simulink model "DeltaWingPlantHGO"  (R2024b)
settings: Solver=VariableStepAuto  StartTime=0.0  StopTime=60  MaxStep=0.01  RelTol=1e-3  EnableMultiTasking=on
InitFcn:
  | global Ba La gamma_a
  | beta0 = 0.4;
  | betap0 = 0;
  | theta10 = -0.018;
  | theta20 = 0.015;
  | mu = 0.1;
  | alpha = 1.5;
  | um = pi;
  | wc = 2*pi/alpha;
  | w0 = wc/mu;
  | theta6 = 0.5;
  | 
  | A = [0 1 0; theta10 theta20 1 ; 0 0 0];
  | B = [0; theta6; 0];
  | C = [1 0 0];
  | 
  | l1 = 3*w0 + theta20;
  | l2 = 3*w0^2 + theta10 + l1*theta20;
  | l3 = w0^3;
  | L = [l1; l2; l3];
  | Ta = 0.04;
  | Tc = 0.1;
  | I = eye(3);
  | gamma = A - L*C;
  | gamma_a = I + Ta*gamma;
  | Ba = Ta*B;
  | La = Ta*L;
  | kp = wc^2+ theta10;
  | kd = 2*wc + theta20;
libraries: simulink x2
settings Model: Creator=Melkamu A  LastModifiedBy=user
settings SolverCC: AlgebraicLoopSolver=TrustRegion
settings DataIOCC: LimitDataPoints=on  SaveFormat=Array  SignalLoggingSaveFormat=ModelDataLogs  ReturnWorkspaceOutputs=off
settings OptimizationCC: InitFltsAndDblsToZero=on  LifeSpan=inf
settings DebuggingCC: SaveWithParameterizedLinksMsg=none  UnderspecifiedInitializationDetection=Classic  MergeDetectMultiDrivingBlocksExec=none  SignalResolutionControl=TryResolveAllWithWarning  SolverPrmCheckMsg=warning  MultiTaskDSMMsg=warning  MultiTaskCondExecSysMsg=none  FcnCallInpInsideContextMsg=warning  UnconnectedInputMsg=warning  UnconnectedOutputMsg=warning  UnconnectedLineMsg=warning  SFUnexpectedBacktrackingDiag=warning  SFNoUnconditionalDefaultTransitionDiag=warning  SFExecutionAtInitializationDiag=none  ArithmeticOperatorsInVariantConditions=warning
settings HardwareCC: ProdBitPerPointer=32  ProdBitPerSizeT=32  ProdBitPerPtrDiffT=32  ProdLargestAtomicFloat=None  ProdIntDivRoundTo=Undefined  ProdEndianess=Unspecified  ProdWordSize=32  ProdHWDeviceType=32-bit Generic
settings ModelReferenceCC: EnableRefExpFcnMdlSchedulingChecks=on  PropagateSignalLabelsOutOfModel=off
settings RTWCC: GPUComputeCapability=3.5  DLArmComputeVersion=19.05
settings CodeAppCC: StateflowObjectComments=on
settings GRTTargetCC: TargetFcnLib=ansi_tfl_tmw.mat  TargetLangStandard=C89/C90 (ANSI)  CombineOutputUpdateFcns=off  GRTInterface=on
settings ConfigComp: CovMetricSettings=dw  CovSaveCumulativeToWorkspaceVar=on  CovSaveSingleToWorkspaceVar=on

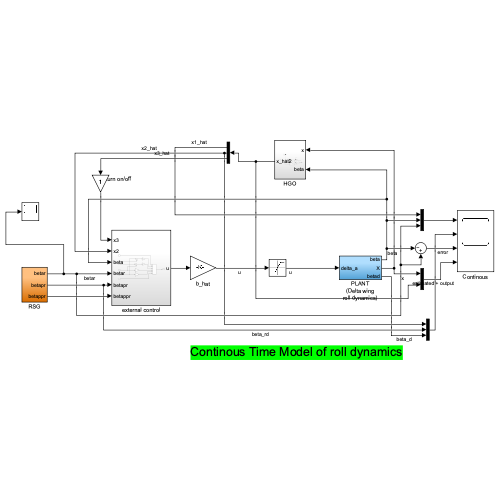
[thumbnail: Simulink's stored preview of the top-level diagram]
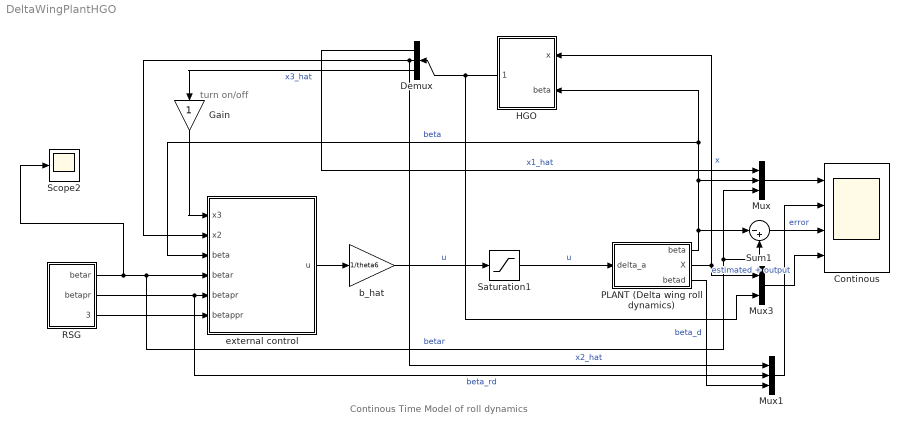
== system DeltaWingPlantHGO ==
  note: turn on/off
  note: Continous Time Model of roll dynamics
  Continous : Scope  NumInputPorts=4
  Demux : Demux  Outputs=3
  Gain : Gain
  HGO : Subsystem
  Mux : Mux  Inputs=3
  Mux1 : Mux  Inputs=3
  Mux3 : Mux  Inputs=2
  PLANT (Delta wing roll dynamics) : Subsystem
  RSG : Subsystem
  Saturation1 : Saturate  UpperLimit=pi  LowerLimit=-pi
  Scope2 : Scope
  Sum1 : Sum  Inputs=|-+
  b_hat : Gain  Gain=1/theta6
  external control : Subsystem
  wires:
  PLANT (Delta wing roll dynamics)/1(beta) -> Sum1/1, HGO/2(beta), external control/3(beta), Mux/2  "beta"
  RSG/1(betar) -> Scope2/1, Sum1/2, Mux/3, external control/4(betar)  "betar"
  RSG/2(betapr) -> Mux1/2, external control/5(betapr)  "beta_rd"
  RSG/3(betappr) -> external control/6(betappr)
  external control/1(u) -> b_hat/1
  Demux/3 -> Gain/1  "x3_hat"
  b_hat/1 -> Saturation1/1  "u"
  Demux/2 -> Mux1/1, external control/2(x2)  "x2_hat"
  Mux/1 -> Continous/1
  Demux/1 -> Mux/1  "x1_hat"
  PLANT (Delta wing roll dynamics)/2(X) -> Mux3/1, HGO/1(x)  "x"
  Mux3/1 -> Continous/4  "estimated + output"
  Sum1/1 -> Continous/3  "error"
  Gain/1 -> external control/1(x3)
  HGO/1(x_hat2) -> Demux/1, Mux3/2
  PLANT (Delta wing roll dynamics)/3(betad) -> Mux1/3  "beta_d"
  Mux1/1 -> Continous/2
  Saturation1/1 -> PLANT (Delta wing roll dynamics)/1(delta_a)  "u"

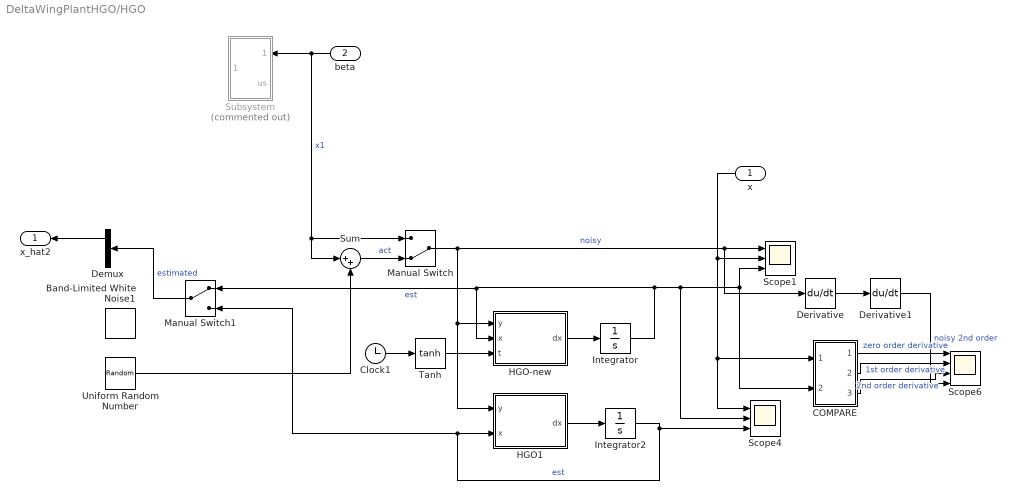
== system DeltaWingPlantHGO/HGO ==
  x : Inport
  beta : Inport  Port=2
  Band-Limited White Noise1 : simulink/Sources/Band-Limited White Noise  Cov=1e-8  Ts=0.001  seed=[23341]
  COMPARE : Subsystem
  Clock1 : Clock
  Demux : Demux  Outputs=[3, 1]
  Derivative : Derivative
  Derivative1 : Derivative
  HGO-new : MATLAB Function  TreatAsAtomicUnit=on
  HGO1 : MATLAB Function  TreatAsAtomicUnit=on
  Integrator : Integrator
  Integrator2 : Integrator
  Manual Switch : ManualSwitch  CurrentSetting=0
  Manual Switch1 : ManualSwitch
  Scope1 : Scope  NumInputPorts=3
  Scope4 : Scope  NumInputPorts=3
  Scope6 : Scope  NumInputPorts=4
  Subsystem : Subsystem  Commented=on
  Sum : Sum  Inputs=|++
  Tanh : Trigonometry  Operator=tanh
  Uniform Random Number : UniformRandomNumber  Minimum=-1e-3  Maximum=1e-3  SampleTime=1e-3
  x_hat2 : Outport
  wires:
  HGO-new/1(dx) -> Integrator/1
  HGO1/1(dx) -> Integrator2/1
  COMPARE/2(Out2) -> Scope6/2  "1st order derivative"
  Sum/1 -> Manual Switch/2  "act"
  beta/1 -> Subsystem/1(beta), Manual Switch/1, Sum/1  "x1"
  x/1 -> Scope1/2, COMPARE/1(act), Scope4/1
  Clock1/1 -> Tanh/1
  Uniform Random Number/1 -> Sum/2
  Tanh/1 -> HGO-new/3(t)
  Derivative1/1 -> Scope6/4  "noisy 2nd order"
  Derivative/1 -> Derivative1/1
  Manual Switch1/1 -> Demux/1  "estimated"
  Integrator/1 -> HGO-new/2(x), Manual Switch1/1, Scope4/2, Scope1/3, COMPARE/2(est)  "est"
  COMPARE/3(Out3) -> Scope6/3  "2nd order derivative"
  COMPARE/1(Out1) -> Scope6/1  "zero order derivative"
  Manual Switch/1 -> Scope1/1, Derivative/1, HGO-new/1(y), HGO1/1(y)  "noisy"
  Integrator2/1 -> Scope4/3, Manual Switch1/2, HGO1/2(x)  "est"
  Demux/1 -> x_hat2/1

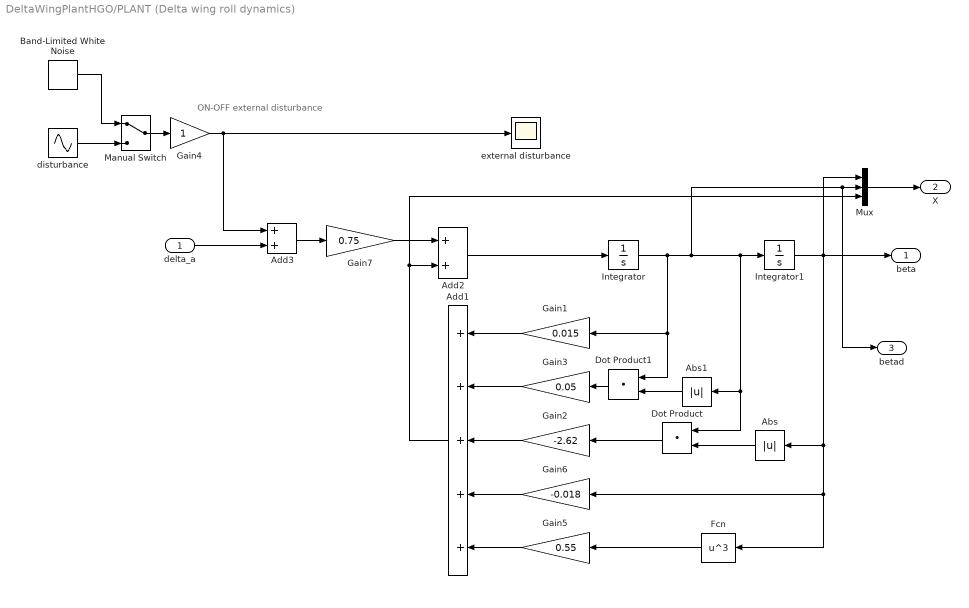
== system DeltaWingPlantHGO/PLANT (Delta wing roll dynamics) ==
  note: ON-OFF external
      | disturbance
  delta_a : Inport
  Abs : Abs  SaturateOnIntegerOverflow=off
  Abs1 : Abs  SaturateOnIntegerOverflow=off
  Add1 : Sum  Inputs=+++++
  Add2 : Sum
  Add3 : Sum
  Band-Limited White Noise : simulink/Sources/Band-Limited White Noise  Cov=[0.1*15]  Ts=15  seed=[23341]
  Dot Product : DotProduct  OutDataTypeStr=Inherit: Inherit via internal rule
  Dot Product1 : DotProduct  OutDataTypeStr=Inherit: Inherit via internal rule
  Fcn : Fcn  Expr=u^3
  Gain1 : Gain  Gain=0.015
  Gain2 : Gain  Gain=-2.62
  Gain3 : Gain  Gain=0.05
  Gain4 : Gain
  Gain5 : Gain  Gain=0.55
  Gain6 : Gain  Gain=-0.018
  Gain7 : Gain  Gain=0.75
  Integrator : Integrator  InitialCondition=betap0
  Integrator1 : Integrator  InitialCondition=beta0
  Manual Switch : ManualSwitch
  Mux : Mux  Inputs=3
  disturbance : Sin  Amplitude=1.5  SampleTime=0
  external disturbance : Scope
  beta : Outport
  X : Outport  Port=2
  betad : Outport  Port=3
  wires:
  Integrator/1 -> Dot Product1/1, Gain1/1, betad/1, Mux/2, Integrator1/1, Dot Product/1, Abs1/1
  Add2/1 -> Integrator/1
  Manual Switch/1 -> Gain4/1
  Band-Limited White Noise/1 -> Manual Switch/1
  disturbance/1 -> Manual Switch/2
  Integrator1/1 -> Mux/1, Gain6/1, Fcn/1, Abs/1, beta/1
  Add1/1 -> Mux/3, Add2/2
  Fcn/1 -> Gain5/1
  Dot Product/1 -> Gain2/1
  Abs/1 -> Dot Product/2
  Abs1/1 -> Dot Product1/2
  Dot Product1/1 -> Gain3/1
  Gain1/1 -> Add1/1
  Gain3/1 -> Add1/2
  Gain2/1 -> Add1/3
  Gain6/1 -> Add1/4
  Gain5/1 -> Add1/5
  Gain4/1 -> external disturbance/1, Add3/1
  Add3/1 -> Gain7/1
  delta_a/1 -> Add3/2
  Gain7/1 -> Add2/1
  Mux/1 -> X/1

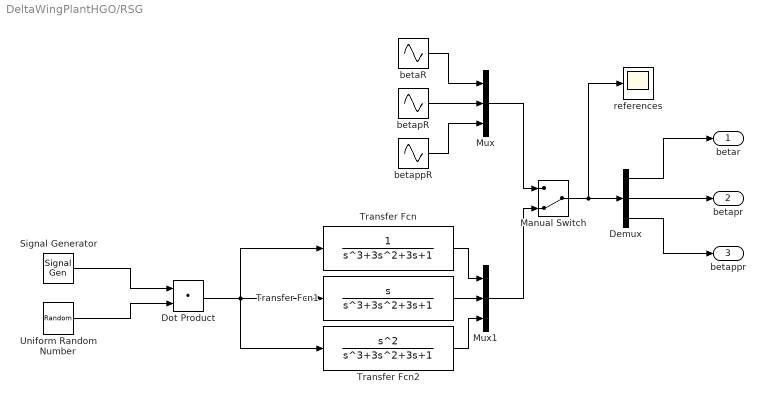
== system DeltaWingPlantHGO/RSG ==
  Demux : Demux  Outputs=3
  Dot Product : DotProduct  OutDataTypeStr=Inherit: Inherit via internal rule
  Manual Switch : ManualSwitch  CurrentSetting=0
  Mux : Mux  Inputs=3
  Mux1 : Mux  Inputs=3
  Signal Generator : SignalGenerator  WaveForm=square  Frequency=0.05
  Transfer Fcn : TransferFcn  Denominator=[1 3 3 1]
  Transfer Fcn1 : TransferFcn  Numerator=[1 0]  Denominator=[1 3 3 1]
  Transfer Fcn2 : TransferFcn  Numerator=[1 0 0]  Denominator=[1 3 3 1]
  Uniform Random Number : UniformRandomNumber  Minimum=-0.8*pi/2  Maximum=0.8*pi/2  SampleTime=10
  betaR : Sin  Frequency=0.5  SampleTime=0
  betapR : Sin  Amplitude=0.5  Frequency=0.5  Phase=pi/2  SampleTime=0
  betappR : Sin  Amplitude=-1*0.5*0.5  Frequency=0.5  SampleTime=0
  references : Scope
  betar : Outport
  betapr : Outport  Port=2
  betappr : Outport  Port=3
  wires:
  betaR/1 -> Mux/1
  betapR/1 -> Mux/2
  betappR/1 -> Mux/3
  Mux/1 -> Manual Switch/1
  Mux1/1 -> Manual Switch/2
  Manual Switch/1 -> Demux/1, references/1
  Demux/2 -> betapr/1
  Demux/1 -> betar/1
  Demux/3 -> betappr/1
  Transfer Fcn/1 -> Mux1/1
  Transfer Fcn1/1 -> Mux1/2
  Transfer Fcn2/1 -> Mux1/3
  Signal Generator/1 -> Dot Product/1
  Uniform Random Number/1 -> Dot Product/2
  Dot Product/1 -> Transfer Fcn2/1, Transfer Fcn/1, Transfer Fcn1/1

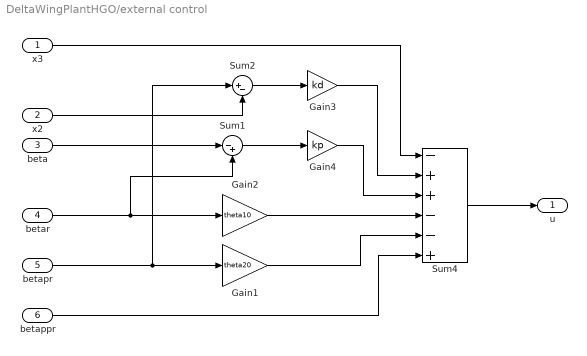
== system DeltaWingPlantHGO/external control ==
  x3 : Inport
  x2 : Inport  Port=2
  beta : Inport  Port=3
  betar : Inport  Port=4
  betapr : Inport  Port=5
  betappr : Inport  Port=6
  Gain1 : Gain  Gain=theta20
  Gain2 : Gain  Gain=theta10
  Gain3 : Gain  Gain=kd
  Gain4 : Gain  Gain=kp
  Sum1 : Sum  Inputs=|-+
  Sum2 : Sum  Inputs=|+-
  Sum4 : Sum  Inputs=-++--+
  u : Outport
  wires:
  x3/1 -> Sum4/1
  beta/1 -> Sum1/1
  betapr/1 -> Gain1/1, Sum2/1
  x2/1 -> Sum2/2
  betar/1 -> Sum1/2, Gain2/1
  Gain3/1 -> Sum4/2
  Sum2/1 -> Gain3/1
  betappr/1 -> Sum4/6
  Sum1/1 -> Gain4/1
  Gain2/1 -> Sum4/4
  Gain4/1 -> Sum4/3
  Sum4/1 -> u/1
  Gain1/1 -> Sum4/5

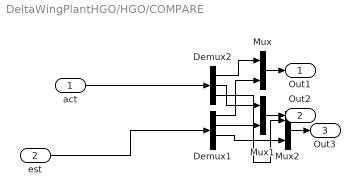
== system DeltaWingPlantHGO/HGO/COMPARE ==
  act : Inport
  est : Inport  Port=2
  Demux1 : Demux
  Demux2 : Demux  Outputs=3
  Mux : Mux  Inputs=2
  Mux1 : Mux  Inputs=2
  Mux2 : Mux  Inputs=2
  Out1 : Outport
  Out2 : Outport  Port=2
  Out3 : Outport  Port=3
  wires:
  est/1 -> Demux1/1
  Demux1/3 -> Mux2/2
  act/1 -> Demux2/1
  Demux2/1 -> Mux/1
  Mux/1 -> Out1/1
  Demux1/2 -> Mux1/2
  Demux1/1 -> Mux/2
  Demux2/2 -> Mux1/1
  Mux2/1 -> Out3/1
  Demux2/3 -> Mux2/1
  Mux1/1 -> Out2/1

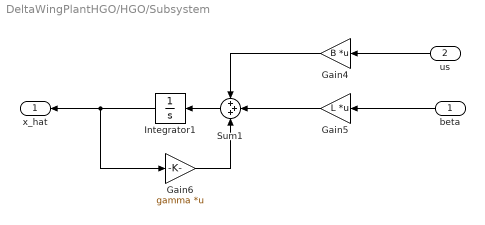
== system DeltaWingPlantHGO/HGO/Subsystem ==
  beta : Inport
  us : Inport  Port=2
  Gain4 : Gain  Gain=B  Multiplication=Matrix(K*u)
  Gain5 : Gain  Gain=L  Multiplication=Matrix(K*u)
  Gain6 : Gain  Gain=gamma  Multiplication=Matrix(K*u)
  Integrator1 : Integrator
  Sum1 : Sum  Inputs=+++
  x_hat : Outport
  wires:
  us/1 -> Gain4/1
  Gain4/1 -> Sum1/1
  Sum1/1 -> Integrator1/1
  Gain5/1 -> Sum1/2
  Integrator1/1 -> x_hat/1, Gain6/1
  Gain6/1 -> Sum1/3
  beta/1 -> Gain5/1

== matlab function DeltaWingPlantHGO/HGO/HGO-new ==
  data: y input; dx output; x input; t input
function dx = fcn(y, x, t)
    % Parameters
    n = 4;                % Order of the observer
    epsilon = 1/200;      % Small gain parameter
    tr = t/10; 
    % Binomial coefficients (for n = 4)
    % ki = nchoosek(n, i)
    k = [4, 6, 4, 1]; 

    e = 1e-5;
    % Initialize output derivative
    dx = zeros(n, 1);
    
    % High-Gain Observer Equations
    dx(1) = x(2) + (k(1)*(tr+e)^1 / epsilon^1) * (y - x(1));
    dx(2) = x(3) + (k(2)*(tr+e)^2 / epsilon^2) * (y - x(1));
    dx(3) = x(4) + (k(3)*(tr+e)^3 / epsilon^3) * (y - x(1));
    dx(4) = (k(4)*(tr+e)^4 / epsilon^4) * (y - x(1));
end

== matlab function DeltaWingPlantHGO/HGO/HGO1 ==
  data: y input; dx output; x input
function dx = fcn(y, x)
    % Parameters
    n = 4;                % Order of the observer
    epsilon = 1/150;      % Small gain parameter
    % tr = 1 ; 
    % Binomial coefficients (for n = 4)
    % ki = nchoosek(n, i)
    k = [4, 6, 4, 1]; 

    % Initialize output derivative
    dx = zeros(n, 1);
    
    % High-Gain Observer Equations
    dx(1) = x(2) + (k(1) / epsilon^1) * (y - x(1));
    dx(2) = x(3) + (k(2) / epsilon^2) * (y - x(1));
    dx(3) = x(4) + (k(3) / epsilon^3) * (y - x(1));
    dx(4) = (k(4) / epsilon^4) * (y - x(1));
end
